simulink model "modelZSB2"  (Simulink 8.3)
settings: Solver=ode4  StartTime=0.0  StopTime=10  FixedStep=0.01  RelTol=1e-3
(part 1 of 3)
settings Model: Creator=Chan Hwaiwing  LastModifiedBy=shubo
settings DataIOCC: SignalLoggingSaveFormat=Dataset
settings DebuggingCC: UnderspecifiedInitializationDetection=Simplified  StateNameClashWarn=none
settings GRTTargetCC: CombineOutputUpdateFcns=on  GRTInterface=off

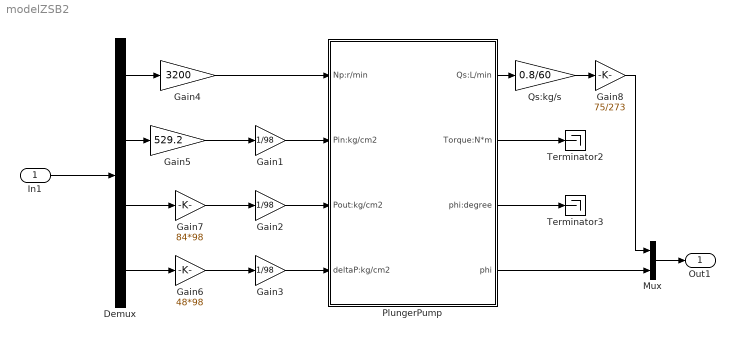
== system modelZSB2 ==
  In1 : Inport
  Demux : Demux
  Gain1 : Gain  Gain=1/98
  Gain2 : Gain  Gain=1/98
  Gain3 : Gain  Gain=1/98
  Gain4 : Gain  Gain=3200
  Gain5 : Gain  Gain=529.2
  Gain6 : Gain  Gain=48*98
  Gain7 : Gain  Gain=84*98
  Gain8 : Gain  Gain=75/273
  Mux : Mux  Inputs=2
  PlungerPump : Subsystem
  Qs:kg/s : Gain  Gain=0.8/60
  Terminator2 : Terminator
  Terminator3 : Terminator
  Out1 : Outport
  wires:
  Gain8/1 -> Mux/1
  PlungerPump/3(phi:degree) -> Terminator3/1
  PlungerPump/1(Qs:L/min) -> Qs:kg/s/1
  PlungerPump/2(Torque:N*m) -> Terminator2/1
  Gain1/1 -> PlungerPump/2(Pin:kg/cm2)
  Gain3/1 -> PlungerPump/4(deltaP:kg/cm2)
  Gain2/1 -> PlungerPump/3(Pout:kg/cm2)
  Demux/1 -> Gain4/1
  Demux/2 -> Gain5/1
  Demux/3 -> Gain7/1
  Demux/4 -> Gain6/1
  Gain5/1 -> Gain1/1
  Gain7/1 -> Gain2/1
  Gain6/1 -> Gain3/1
  Gain4/1 -> PlungerPump/1(Np:r/min)
  PlungerPump/4(phi) -> Mux/2
  Mux/1 -> Out1/1
  Qs:kg/s/1 -> Gain8/1
  In1/1 -> Demux/1

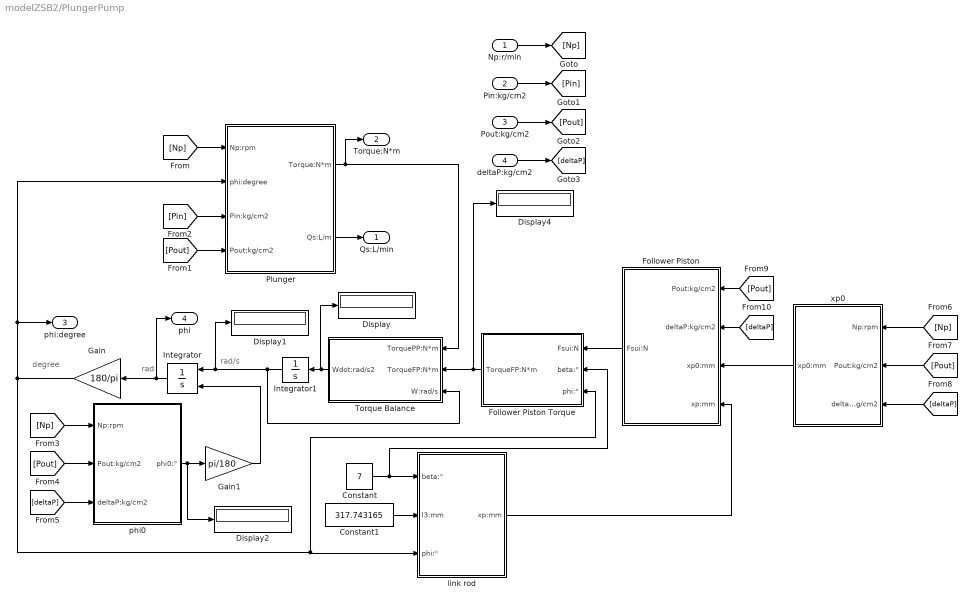
== system modelZSB2/PlungerPump ==
  note: rad/s
  note: rad
  note: degree
  Np:r/min : Inport
  Pin:kg/cm2 : Inport  Port=2
  Pout:kg/cm2 : Inport  Port=3
  deltaP:kg/cm2 : Inport  Port=4
  Constant : Constant  Value=7
  Constant1 : Constant  Value=317.743165
  Display{,1..2,4} (4 alike) : Display
  Follower Piston : Subsystem
  Follower Piston Torque : Subsystem
  Gain : Gain  Gain=180/pi
  Gain1 : Gain  Gain=pi/180
  Integrator : Integrator  InitialConditionSource=external  LimitOutput=on  UpperSaturationLimit=14.8/180*pi  LowerSaturationLimit=0
  Integrator1 : Integrator  InitialCondition=1
  Plunger : Subsystem
  Torque Balance : Subsystem
  link rod : Subsystem
  phi0 : Subsystem
  xp0 : Subsystem
  Qs:L/min : Outport
  Torque:N*m : Outport  Port=2
  phi:degree : Outport  Port=3
  phi : Outport  Port=4
  wires:
  Np:r/min/1 -> [Np]
  [Np] -> Plunger/1(Np:rpm)
  Pin:kg/cm2/1 -> [Pin]
  Pout:kg/cm2/1 -> [Pout]
  [Pin] -> Plunger/3(Pin:kg/cm2)
  deltaP:kg/cm2/1 -> [deltaP]
  [Pout] -> Plunger/4(Pout:kg/cm2)
  Gain/1 -> link rod/3(phi:°), Follower Piston Torque/3(phi:°), phi:degree/1, Plunger/2(phi:degree)
  Integrator/1 -> phi/1, Gain/1
  Integrator1/1 -> Torque Balance/3(W:rad/s), Display1/1, Integrator/1
  Torque Balance/1(Wdot:rad/s2) -> Display/1, Integrator1/1
  Follower Piston Torque/1(TorqueFP:N*m) -> Display4/1, Torque Balance/2(TorqueFP:N*m)
  Follower Piston/1(Fsui:N) -> Follower Piston Torque/1(Fsui:N)
  phi0/1(phi0:°) -> Display2/1, Gain1/1
  Gain1/1 -> Integrator/2
  [Np] -> phi0/1(Np:rpm)
  [Pout] -> phi0/2("Pout:kg/cm2 ")
  [deltaP] -> phi0/3(deltaP:kg/cm2)
  Constant/1 -> Follower Piston Torque/2(beta:°), link rod/1(beta:°)
  Constant1/1 -> link rod/2(l3:mm)
  link rod/1(xp:mm) -> Follower Piston/4(xp:mm)
  [Pout] -> Follower Piston/1(Pout:kg/cm2)
  [deltaP] -> Follower Piston/2(deltaP:kg/cm2)
  Plunger/1(Torque:N*m) -> Torque Balance/1(TorquePP:N*m), Torque:N*m/1
  Plunger/2(Qs:L/m) -> Qs:L/min/1
  xp0/1(xp0:mm) -> Follower Piston/3(xp0:mm)
  [Np] -> xp0/1(Np:rpm)
  [Pout] -> xp0/2("Pout:kg/cm2 ")
  [deltaP] -> xp0/3(deltaP:kg/cm2)

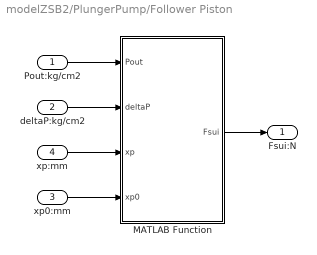
== system modelZSB2/PlungerPump/Follower Piston ==
  Pout:kg/cm2 : Inport
  deltaP:kg/cm2 : Inport  Port=2
  xp0:mm : Inport  Port=3
  xp:mm : Inport  Port=4
  MATLAB Function : MATLAB Function  TreatAsAtomicUnit=on
  Fsui:N : Outport
  wires:
  Pout:kg/cm2/1 -> MATLAB Function/1(Pout)
  deltaP:kg/cm2/1 -> MATLAB Function/2(deltaP)
  xp:mm/1 -> MATLAB Function/3(xp)
  xp0:mm/1 -> MATLAB Function/4(xp0)
  MATLAB Function/1(Fsui) -> Fsui:N/1

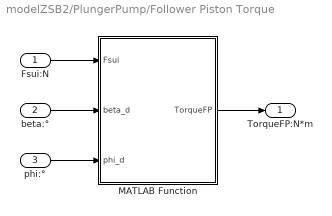
== system modelZSB2/PlungerPump/Follower Piston Torque ==
  Fsui:N : Inport
  beta:° : Inport  Port=2
  phi:° : Inport  Port=3
  MATLAB Function : MATLAB Function  TreatAsAtomicUnit=on
  TorqueFP:N*m : Outport
  wires:
  Fsui:N/1 -> MATLAB Function/1(Fsui)
  beta:°/1 -> MATLAB Function/2(beta_d)
  phi:°/1 -> MATLAB Function/3(phi_d)
  MATLAB Function/1(TorqueFP) -> TorqueFP:N*m/1

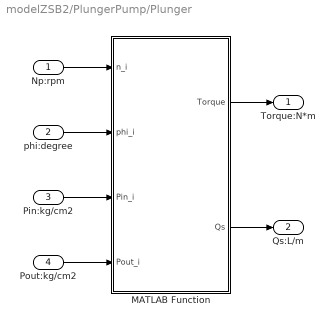
== system modelZSB2/PlungerPump/Plunger ==
  Np:rpm : Inport
  phi:degree : Inport  Port=2
  Pin:kg/cm2 : Inport  Port=3
  Pout:kg/cm2 : Inport  Port=4
  MATLAB Function : MATLAB Function  TreatAsAtomicUnit=on
  Torque:N*m : Outport
  Qs:L/m : Outport  Port=2
  wires:
  Np:rpm/1 -> MATLAB Function/1(n_i)
  Pout:kg/cm2/1 -> MATLAB Function/4(Pout_i)
  Pin:kg/cm2/1 -> MATLAB Function/3(Pin_i)
  phi:degree/1 -> MATLAB Function/2(phi_i)
  MATLAB Function/2(Qs) -> Qs:L/m/1
  MATLAB Function/1(Torque) -> Torque:N*m/1

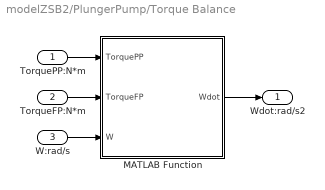
== system modelZSB2/PlungerPump/Torque Balance ==
  TorquePP:N*m : Inport
  TorqueFP:N*m : Inport  Port=2
  W:rad/s : Inport  Port=3
  MATLAB Function : MATLAB Function  TreatAsAtomicUnit=on
  Wdot:rad/s2 : Outport
  wires:
  W:rad/s/1 -> MATLAB Function/3(W)
  TorqueFP:N*m/1 -> MATLAB Function/2(TorqueFP)
  TorquePP:N*m/1 -> MATLAB Function/1(TorquePP)
  MATLAB Function/1(Wdot) -> Wdot:rad/s2/1

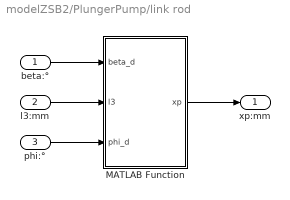
== system modelZSB2/PlungerPump/link rod ==
  beta:° : Inport
  l3:mm : Inport  Port=2
  phi:° : Inport  Port=3
  MATLAB Function : MATLAB Function  TreatAsAtomicUnit=on
  xp:mm : Outport
  wires:
  l3:mm/1 -> MATLAB Function/2(l3)
  MATLAB Function/1(xp) -> xp:mm/1
  phi:°/1 -> MATLAB Function/3(phi_d)
  beta:°/1 -> MATLAB Function/1(beta_d)

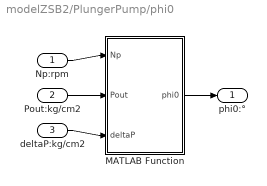
== system modelZSB2/PlungerPump/phi0 ==
  Np:rpm : Inport
  "Pout:kg/cm2 " : Inport  Port=2
  deltaP:kg/cm2 : Inport  Port=3
  MATLAB Function : MATLAB Function  TreatAsAtomicUnit=on
  phi0:° : Outport
  wires:
  Np:rpm/1 -> MATLAB Function/1(Np)
  "Pout:kg/cm2 "/1 -> MATLAB Function/2(Pout)
  deltaP:kg/cm2/1 -> MATLAB Function/3(deltaP)
  MATLAB Function/1(phi0) -> phi0:°/1

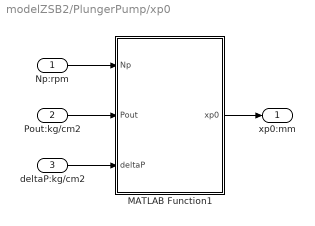
== system modelZSB2/PlungerPump/xp0 ==
  Np:rpm : Inport
  "Pout:kg/cm2 " : Inport  Port=2
  deltaP:kg/cm2 : Inport  Port=3
  MATLAB Function1 : MATLAB Function  TreatAsAtomicUnit=on
  xp0:mm : Outport
  wires:
  "Pout:kg/cm2 "/1 -> MATLAB Function1/2(Pout)
  Np:rpm/1 -> MATLAB Function1/1(Np)
  deltaP:kg/cm2/1 -> MATLAB Function1/3(deltaP)
  MATLAB Function1/1(xp0) -> xp0:mm/1

== matlab function PlungerPump/Plunger/MATLAB Function ==
  data: n_i input double; Torque output double; phi_i input double; Pin_i input double; Pout_i input double; Qs output double
function [ Torque, Qs] = Plunger_Pump(n_i, phi_i, Pin_i, Pout_i)
% All length unit: mm
% ********** Technical Specifications **************
% i=0.2318,i=n_H/n_P;
% Tin:-40℃~+135℃;
% Pin:0.412~0.892MPa;
% Pout:4.138~8.277MPa;
% Qmax=11820L/h;
% Follower Piston deltaP:1.38~4.34MPa;
% Safety Valve open pressure:12.4MPa;
% m_pump=20.7kg;
% **************************************************
% *********** Parameter Nomenclature ***************
% n_i:Pump Speed;
% phi_i: Pump Swash plate angle;
% Pin_i:Pump inlet Pressure,unit,kg/cm2;
% Pout_i:Pump outlet Pressure,unit,kg/cm2;
% etaV:Pump volumetric efficiency;
% z:the number of plungers;
% a:定尺寸，柱塞轴线交点O到斜盘锥面顶点A距离；
% c:斜盘转轴A与斜盘球面中心O1的距离；
% rcphi:柱塞头部球面半径；
% theta: install angle;
% d1:柱塞底面内径；
% dzr:柱塞中部内径；
% Smax:piston max travel distance at swash angle phi;
% qL1:a theoretical amount of supplied fuel of one piston at one rotation,cm3/r;
% QL: a actual amount of supplied fuel of Pump,L/min;
% Torque:all plungers on swashplate mean torque;Clockwise is positive;
%% Correction Factor
% CF = 1.14;
CF = 1.00;
%% ****** Plunger Centroid Calculate BEGIN *****
dz = (23.7820+23.8074+23.8328+23.8582+23.8836)*CF/5;
d11 = 22.6*CF;
d12 = 19*CF;
l1 = 2.9*CF;
V1a = pi/3*l1*(d11*d11/4+d12*d12/4+d11*d12/4);
V1b = pi/4*dz*dz*l1;
V1 = V1b-V1a;

lr = 48.8*CF;
l2 = lr-l1;
d2 = 19*CF;
V2 = pi/4*(dz*dz-d2*d2)*l2;

l3 = (5.5-3.2)/2/tan(60*pi/180)*CF;
d31 = 5.5*CF;
d32 = 3.2*CF;
V3a = pi/3*l3*(d31*d31/4+d32*d32/4+d31*d32/4);
V3b = pi/4*dz*dz*l3;
V3 = V3b-V3a;

l4 = (51.5-48.8)*CF-l3;
d4 = 3.2*CF;
V4 = pi/4*(dz*dz-d4*d4)*l4;

l5 = 5/2*sin(45*pi/180)*CF;
d51 = dz;
d52 = dz-2*5/2*cos(45*pi/180)*CF;
d5 = 3.2*CF;
V5a = pi/4*d5*d5*l5;
V5b = pi/3*l5*(d51*d51/4+d52*d52/4+d51*d52/4);
V5 = V5b-V5a;

l6 = 7.4/2*sin(20*pi/180)*CF;
d61 = d52;
d62 = 12.8*CF;
d6 = 3.2*CF;
V6a = pi/4*d6*d6*l6;
V6b =  pi/3*l6*(d61*d61/4+d62*d62/4+d61*d62/4);
V6 = V6b-V6a;

l7 = (17.2-16)*CF;
d71 = 12.8*CF;
d72 = 3.2*CF;
V7 = pi/4*(d71*d71-d72*d72)*l7;

SR = 19.05/2*CF;
d8 = 3.2*CF;
d81 = 12.8*CF;
d82 = 5*CF;
l81 = SR-sqrt(SR*SR-d81*d81/4);
l82 = SR-sqrt(SR*SR-d82*d82/4);
l8 = 2*SR - l81 - l82;
V81 = pi/3*l81*l81*(3*SR-l81);
V82 = pi/3*l82*l82*(3*SR-l82);
VS8 = 4/3*pi*SR*SR*SR;
V83 = pi/4*d8*d8*l8;
V8 = VS8 - V81 - V82 - V83;

% V = V1+V2+V3+V4+V5+V6+V7+V8;

X1a = l1*(d11*d11/4+2*d11/2*d12/2+3*d12*d12/4)/4/(d11*d11/4+d11/2*d12/2+d12*d12/4);
X1b = l1/2;
X1 = (V1b*X1b-V1a*X1a)/(V1b-V1a);

X2p = l2/2;
X2 = X2p+l1;

X3a = l3*(d31*d31/4+2*d31/2*d32/2+3*d32*d32/4)/4/(d31*d31/4+d31/2*d32/2+d32*d32/4);
X3b = l3/2;
X3p = (V3b*X3b-V3a*X3a)/(V3b-V3a);
X3 = X3p+lr;

X4p = l4/2;
X4 = X4p+48.8*CF+l3;

X5a = l5/2;
X5b = l5*(d51*d51/4+2*d51/2*d52/2+3*d52*d52/4)/4/(d51*d51/4+d51/2*d52/2+d52*d52/4);
X5p = (V5b*X5b-V5a*X5a)/(V5b-V5a);
X5 = X5p+51.5*CF;

X6a = l6/2;
X6b = l6*(d61*d61/4+2*d61/2*d62/2+3*d62*d62/4)/4/(d61*d61/4+d61/2*d62/2+d62*d62/4);
X6p = (V6b*X6b-V6a*X6a)/(V6b-V6a);
X6 = X6p+51.5*CF+l5;

X7p = l7/2;
X7 = X7p+51.5*CF+l5+l6;

X8a = SR-3*(2*SR-l81)*(2*SR-l81)/4/(3*SR-l81);
X8b = SR+3*(2*SR-l82)*(2*SR-l82)/4/(3*SR-l82);
X8c = SR;
X8d = (VS8*X8c-V81*X8a-V82*X8b)/(VS8-V81-V82)-l81;
X8e = l8/2;
X8p = ((VS8-V81-V82)*X8d - V83*X8e)/(VS8-V81-V82-V83);

X8 = X8p+(72.62-16)*CF;

Xc = (V1*X1+V2*X2+V3*X3+V4*X4+V5*X5+V6*X6+V7*X7+V8*X8)/(V1+V2+V3+V4+V5+V6+V7+V8);

k = 63.2*CF-Xc;

mz = 0.1006*CF;

%% ****** Plunger Centroid Calculate END *********
%% ****** Plunger Kinematics Calculate BEGIN *****
R = 266.7*CF;
theta = 10*pi/180;
dz = (23.7820+23.8074+23.8328+23.8582+23.8836)*CF/5;
% h = 19.05*16/22*0.1*CF;
h = 17*0.45/0.6*CF;
etaV = 0.95;
z = 7;
a = R/cos(theta);
c = a;
phi = phi_i*pi/180;
R0 = sqrt(c*c+a*a-2*c*a*cos(phi));
tau = atan((cos(phi)-a/c)/sin(phi));
% tau_d = tau*180/pi;
L = R-h;
lambda = R0/L;
A1 = -cos(theta)*sin(tau);
B1 = -sin(theta)*cos(tau);
D = 1+lambda*A1-lambda*lambda*(1-A1*A1-B1*B1/2)/2;
E = lambda*B1*(1+lambda*A1);
F = lambda*lambda*B1*B1;
% rou = L*(D+E*cos(alpha)+F*cos(2*alpha)/4);
Smax = -2*L*E;
qL = pi/4*dz*dz*Smax*z*1e-6;
QL = qL*n_i;
Qs = QL*etaV;
%% ****** Plunger Kinematics Calculate END *****
%% ****** Plunger Force and total Torque Calculation BEGIN ******
r1 = 35/2*CF;
r2 = 57.8*CF*cos(15*pi/180);
rou_fuel = 775;
kesi = 0.75;
Kt = (70.27-9.11)/((77.3-50.2)-(77.3-73.8));
l01 = 77.3*CF;
b = (82.55/2/sin(10*pi/180)-69)*CF;
e1 = 7.2*CF;
e2 = 2.5*CF;
e3 = (63.2-48.8)*CF;
omiga = pi*n_i/30;

% alpha_d = alpha*180/pi;
Pin = Pin_i*0.098;%Mpa
Pout = Pout_i*0.098;%Mpa

M = ceil(360/z);
MA2=zeros(M+1,z+2);
for i=0:1:M
    if (i == M)
        alpha2_d = 360/z;
    else
        alpha2_d = i;
    end
    MA2(i+1,1) = alpha2_d;
    all = 0;
    P = 0;
    for j=0:1:(z-1)
        alpha_d = alpha2_d+j*360/z;
        alpha = alpha_d*pi/180;
        rou = L*(D+E*cos(alpha)+F*cos(2*alpha)/4);
        % S = L*(E*cos(alpha)-E+F*cos(2*alpha)/4-F/4);
        %v  = -L*omiga*(E*sin(alpha)+F*sin(2*alpha)/2);
        acc = -L*omiga*omiga*(E*cos(alpha)+F*cos(2*alpha));
        if (alpha_d<=180)
            P = Pin;
        elseif(alpha_d>180&&alpha_d<360)
            P = Pout;
        elseif(alpha_d>=360&&alpha_d<540)
            P = Pin;
        elseif(alpha_d>=540&&alpha_d<=720) 
            P = Pout;
        end
        % 柱塞腔内的油压力
        dzr = 3.2*CF;
        Fu1 = pi/4*(dz*dz-dzr*dzr)*1e-6*P*1e6;
        % 转子腔内的油压力
        d_yaotou = 17*1.0/0.6*CF;
        phi2 = acos((rou*rou+L*L-R0*R0)/2/rou/L);
        Pz = Pin+rou_fuel/2*kesi*(r2*r2-r1*r1)*1e-6*omiga*omiga*1e-6;%--转子腔油压，/Mpa
        Fu2 = pi/4*(d_yaotou*d_yaotou-(dz*dz-dzr*dzr)*cos(phi2))*1e-6*Pz*1e6;%--fuel pressure force,/N
        % plunger spring force
        Ft = Kt*(b+e1+l01+e2+e3)-Kt*rou;%--spring force,/N
        % New Add Cage spring force
        l02 = 56.6;
        Kt2 = 44.39/(56.6-14.3);
        % washer thickness
        t2 = (1.05+1.10+1.20+1.30+1.35+1.40+1.55+1.60+1.65+1.80+1.95)/11;
        B2 = 19.7+t2+6.4-12.8;
        Ft2 = Kt2*(l02 - B2);
        Ft2f = Ft2/cos(phi);
        theta_f = 10*pi/180;
        Ft2i = Ft2f/cos(theta_f)/z;
        % plunger centrifugal force
        FL = mz*omiga*omiga*(rou-k)*1e-3*sin(theta);%/N
        FLz = FL*sin(theta);
        %FLy = FL*cos(theta);%--Centrifugal force+Ft2i
        % relative motion inertial force
        Fg = -mz*acc*1e-3;%--inertia force
        % coriolis inertia force
        % ak = 2*omiga*v*sin(theta)
        % Fk = -mak;
        FsigmaZZ = Fu1+Ft+FLz+Fg;%--plinger axial total force
        FA = FsigmaZZ/cos(phi2)+Fu2+Ft2i;
        A11 = ((a+R0*sin(tau))*sin(theta)*cos(alpha)-R0*cos(tau)*cos(theta))/L;%--total force, one piston, on plate
        h1 = a*R0*cos(tau)/L;
        lt = A11*rou+h1;
        MA = FA*lt*1e-3;
        MA2(i+1,j+2) = MA;%--total torque, one piston
        all = all+MA2(i+1,j+2);
    end
    MA2(i+1,z+2) = all;
end
%% ****** Plunger Force Calculation END ********
%% ****** Plunger mean Torque Calculation BEGIN ******
%%%**** in total torque figure,x-axis represents alpha,20°correspond to 10mm; y-axis represents total torque,20N*m correspond to 10mm; 
sum=0;
kx = 10/20;
ky = 10/20;
for i2=1:1:M
    x1 = MA2(i2,1);
    y1 = MA2(i2,z+2);
    x2 = MA2(i2+1,1);
    y2 = MA2(i2+1,z+2);
    if(y1*y2>=0)
        S = 0.5*(y1*ky+y2*ky)*(x2-x1)*kx;
    else
        x0 = x1-y1/(y2-y1)*(x2-x1);
        S = 0.5*y1*ky*(x0-x1)*kx+0.5*y2*ky*(x2-x0)*kx;
    end
    sum = sum+S;
end
MAa = sum*(1/ky)/(360/z*kx);
Torque = MAa * (-1);
%% ****** Plunger mean Torque Calculation END ******
end

== matlab function PlungerPump/link rod/MATLAB Function ==
  data: beta_d input double; l3 input double; phi_d input double; xp output double
function xp = fcn(beta_d,l3,phi_d)
% l0:mm
% l1:mm
% l2:mm
% l3:mm
% l4:mm
phi = phi_d*pi/180;
beta = beta_d*pi/180;
% l0 = 78.6;
l0 = 17*2.3/0.6;
l1 = 17*2.48/0.6;
l2 = 42.9;
% l3 = 178-14.2+147.4+6.6*17/6;
% l3 = 313.7765;
l4 = 165.3;
xp = l3+l0*sin(phi+beta)-l4-sqrt(l2*l2-(l1-l0*cos(phi+beta))^2);
end

== matlab function PlungerPump/Torque Balance/MATLAB Function ==
  data: TorquePP input double; Wdot output double; TorqueFP input double; W input double
function Wdot = fcn(TorquePP, TorqueFP, W)
%  TorqueOut  unit : Nm
% TorqueFP   unit : Nm
%  W  unit:  radian /s
% J unit: kg.m2
% J =0.0034*1;
J =0.34*0.1;  
%Wdot = ( TorquePP + TorqueFP - 0.2*sign(W) - 0.1*W*30/pi )/ J;
% Wdot = ( TorqueOut + TorqueFP - 0.2 - 0.1*W*30/pi )/ J;
%Wdot = ( TorqueOut - TorqueFP - 0.2 )/ J;
% Wdot = ( TorquePP + TorqueFP )/ J;
% Wdot = ( TorquePP + TorqueFP  - 0.1*W*30/pi )/ J;
Wdot = ( TorquePP + TorqueFP  - 0.1*W*30/pi )/ J;
end

== matlab function PlungerPump/Follower Piston Torque/MATLAB Function ==
  data: Fsui input double; TorqueFP output double; beta_d input double; phi_d input double
function TorqueFP = fcn(Fsui,beta_d,phi_d)
% l0:mm
% l1:mm
% l2:mm
phi = phi_d*pi/180;
beta = beta_d*pi/180;
l0 = 17*2.3/0.6;
l1 = 17*2.48/0.6;
l2 = 42.9;
delta = asin((l1-l0*cos(phi+beta))/l2);
M_Fsui = Fsui/cos(delta)*cos(delta-phi-beta)*l0*0.001;
TorqueFP = M_Fsui*1;
end

== matlab function PlungerPump/Follower Piston/MATLAB Function ==
  data: Pout input double; Fsui output double; deltaP input double; xp input double; xp0 input double
function Fsui = fcn(Pout,deltaP,xp,xp0)
%  Pout unit:kg/cm2
%  deltaP unit:kg/cm2
%  deltaSh unit:mm
%  all length unit:mm
%  Fsui  unit  :  N
D1 = 33.26;%mm
D2 = 17;%mm
D3 = 19.8;%mm
Kt1 = (1421-754.6)/((139.7-101.9)-(139.7-119.6));%N/mm
Kt2 = (1754-1313)/((158-96.8)-(158-114.6));%N/mm
Pleft = Pout*0.098*1e6;%Pa
Pright = Pleft-deltaP*0.098*1e6;%Pa
Fleft = Pleft*pi*(D1^2-D2^2)/4*1e-6;%N
Fright = Pright*pi*(D1^2-D3^2)/4*1e-6;%N
Fs = (Kt1+Kt2)*(139.7-xp+xp0);
Fsui=Fs+Fright-Fleft;
end
